simulink model "test1_diff_2016b"  (R2016b)
settings: Solver=VariableStepAuto  StartTime=0.0  StopTime=10.0  RelTol=1e-3
settings Model: Creator=monika  LastModifiedBy=gm

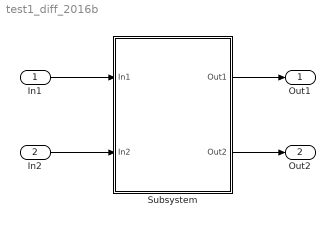
== system test1_diff_2016b ==
  In1 : Inport
  In2 : Inport  Port=2
  Subsystem : Subsystem
  Out1 : Outport
  Out2 : Outport  Port=2
  wires:
  Subsystem/1(Out1) -> Out1/1
  In1/1 -> Subsystem/1(In1)
  In2/1 -> Subsystem/2(In2)
  Subsystem/2(Out2) -> Out2/1

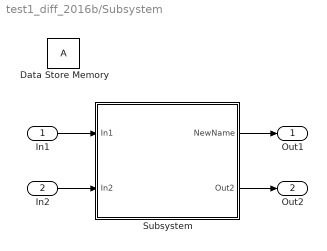
== system test1_diff_2016b/Subsystem ==
  In1 : Inport
  In2 : Inport  Port=2
  Data Store Memory : DataStoreMemory  ReadBeforeWriteMsg=warning  WriteAfterWriteMsg=warning  WriteAfterReadMsg=warning  ShowAdditionalParam=off
  Subsystem : Subsystem
  Out1 : Outport
  Out2 : Outport  Port=2
  wires:
  In1/1 -> Subsystem/1(In1)
  In2/1 -> Subsystem/2(In2)
  Subsystem/1(NewName) -> Out1/1
  Subsystem/2(Out2) -> Out2/1

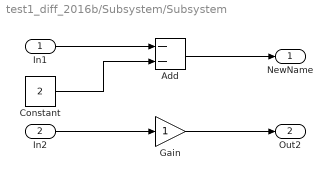
== system test1_diff_2016b/Subsystem/Subsystem ==
  In1 : Inport
  In2 : Inport  Port=2
  Add : Sum  Inputs=--
  Constant : Constant  Value=2
  Gain : Gain
  NewName : Outport
  Out2 : Outport  Port=2
  wires:
  In1/1 -> Add/1
  Add/1 -> NewName/1
  Constant/1 -> Add/2
  In2/1 -> Gain/1
  Gain/1 -> Out2/1
